simulink library "pv_desoto"  (R2018b)
settings: Solver=VariableStepAuto  StartTime=0.0  StopTime=10.0  RelTol=1e-3
undefined symbols (not defined in the file): Davies, Hay, path_carnot
libraries: carnot x4
settings Model: Creator=P41573  LastModifiedBy=P41573
settings SFSimCC: SimUseLocalCustomCode=off
settings RTWCC: RTWUseLocalCustomCode=off
settings CodeAppCC: StateflowObjectComments=on

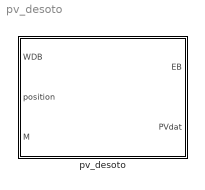
== system pv_desoto ==
  pv_desoto : Subsystem  mask(configurated PV Panel){PathName=fullfile(path_carnot('libsl'), 'Source', 'Electric_Generator', 'pv_desoto', 'parameter_set'), FileName='CEC_sungen_SG-HN100-GG.mat', userPath=on, userParam=on, IL_ref=1.656, alpha_sc=0.001782, a_ref=3.7943, Rs_ref=7.904, Rsh_ref=360.51, I0_ref=1.353e-11, Sref=1000, Tref=25, EgRef=1.121, dEgdT=-0.0002677, KbAngles=[0:5:90], Kb=[1 1 0.9999 0.9996 0.9991 0.9982 0.9965 0.9935 0.9886 0.9807 0.9678 0.9473 0.9148 0.8638 0.7846 0.6644 0.4907 0.2599 0], Kd=0.91, TypeMount=<propagated>, E0=1000, dTc=3, a=-3.348, b=-0.0914, TimeConstant=300, tini=20, ms=1, mp=1}
      mask prompts: PathName "Path"; FileName "Parameter set"; userPath "Edit path and name of parameter set"; userParam "User defined parameters"; IL_ref "reference photo current [A]"; alpha_sc "temperature coef. for Isc [-]"; a_ref "modified diode ideality factor"; Rs_ref "reference serial resistance"; Rsh_ref "reference shunt resistance"; I0_ref "reference saturation current [A]"; Sref "reference irradiance [W/m2]"; Tref "reference cell temperature [°C]"; EgRef "reference band gap [eV]"; dEgdT "temperature dependance of band gap [1/K]"; KbAngles "Kb: angles for longitudinal and transversal IAM [degree]"; Kb "Kb : incident angle modifier beam radiation"; Kd "Kd : Incidence angle modifier diffuse radiation"; TypeMount "Panel type / Mounting Option"; E0 "Reference Irradiation for deltaT (W/m2)"; dTc "SAPM Parameter - deltaT"; a "SAPM Parameter a"; b "SAPM Parameter - b"; TimeConstant "time constant  [s] - (not used)"; tini "initial cell temperature [°C] -(not used)"; ms "Number of modules in series"; mp "Number of modules in parallel"
      mask help:
      | PVPMC (PV-Lib) Single Diode equivalent Model with Sandia temperature model.
      | Parameter tables according to CeC SAMLIB.
      mask init:
      | % [ok, param] = CarnotCallbacks_PvDesotoConf('SetParameters',gcbh,PathName,FileName);
      mask Help: web(fullfile(path_carnot('help'),'pv_desoto.html'),'-helpbrowser')
      mask Callback userPath: [ok, param] = CarnotCallbacks_PvDesoto('UserEdit',gcbh);
      mask Callback userParam: [ok, param] = CarnotCallbacks_PvDesoto('UserEdit',gcbh);
      mask TypeOptions IL_ref: pvl_DeSoto_Sam/IL_ref
      mask TypeOptions alpha_sc: pvl_DeSoto_Sam/alpha_isc
      mask TypeOptions a_ref: pvl_DeSoto_Sam/a_ref
      mask TypeOptions Rs_ref: pvl_DeSoto_Sam/Rs_ref
      mask TypeOptions Rsh_ref: pvl_DeSoto_Sam/Rsh_ref
      mask TypeOptions I0_ref: pvl_DeSoto_Sam/I0_ref
      mask TypeOptions Sref: pvl_DeSoto_Sam/Sref
      mask TypeOptions Tref: pvl_DeSoto_Sam/Tref
      mask TypeOptions EgRef: pvl_DeSoto_Sam/EgRef
      mask TypeOptions dEgdT: pvl_DeSoto_Sam/dEgdT
      mask TypeOptions KbAngles: IAM_Table/angle
      mask TypeOptions Kb: IAM_Table/Kb
      mask TypeOptions Kd: IAM_Table/Kd
      mask TypeOptions TypeMount: <propagated> | Glass/cell/glass - Open rack | Glass/cell/glass - Close roof mount | Glass/cell/polymer sheet - Open rack | Glass/cell/polymer sheet - Insulated back | Polymer/thin-film/steel - Open rack
      mask Callback TypeMount: [ok, param] = CarnotCallbacks_PvDesoto('SetParameters',gcbh);
      mask DialogControl ParameterGroupVar Prompt: Picking a parameter set
      mask DialogControl Control2 Prompt: Carnot public data
      mask DialogControl Control2 Callback: [ok, file] = CarnotCallbacks_PvDesoto('GetFilename',gcbh,'public');
      mask DialogControl Control3 Prompt: Carnot internal data
      mask DialogControl Control3 Callback: [ok, file] = CarnotCallbacks_PvDesoto('GetFilename',gcbh,'internal');
      mask DialogControl Control4 Prompt: Selected path
      mask DialogControl Control4 Callback: [ok, file] = CarnotCallbacks_PvDesoto('GetFilename',gcbh,'selected');
      mask DialogControl Container4 Prompt: Model Parameters
      mask DialogControl Container10 Prompt: PV Panel
      mask DialogControl Container9 Prompt: Optics
      mask DialogControl Container14 Prompt: Temperature Model
      mask DialogControl Container15 Prompt: Array
      mask Display:
      | % user defined picture file
      | picfile = fullfile(path_carnot('intlibsl'), ...
      |         'Source','Electric_Generator','pv_desoto','parameter_set', ...
      |         'pv_desoto.jpg');
      | pic = false;
      | if ~BlockIsInCarnotLibrary    % if not located in library any more
      |     if exist(picfile,'file') % show internal picture if defined
      |         image(imread(picfile), [0.2, 0, 0.6, 1])
      |         set_param(gcb, 'BackgroundColor', 'White')
      |         pic = true;
      |     end
      | end
      | if ~pic    % show public picture
      |     disp('PV-Model\nDesoto')
      |     set_param(gcb, 'BackgroundColor', '[0.5,0.5,1]')
      | end

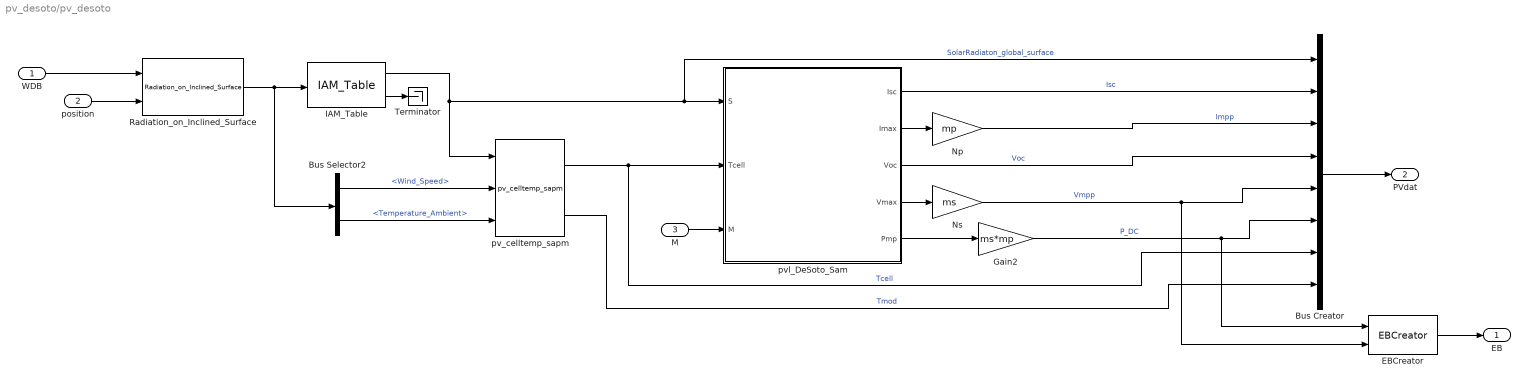
== system pv_desoto/pv_desoto ==
  WDB : Inport
  position : Inport  Port=2
  M : Inport  Port=3
  Bus Creator : BusCreator  Inputs=8
  Bus Selector2 : BusSelector  OutputSignals=Wind_Speed,Temperature_Ambient
  EBCreator : carnot/Basic/Electric/EBCreator  Inport_ID=off  Inport_f=off  Inport_v1=on  Inport_p1=on  Inport_pf1=off  Inport_v2=off  Inport_p2=off  Inport_pf2=off  Inport_v3=off  Inport_p3=off  Inport_pf3=off  ID=2  f=0  v1=0  p1=1e5  pf1=1  v2=0  p2=0  pf2=0  v3=0  p3=0  pf3=0  Annotation_ID=off  Annotation_f=off  Annotation_v1=off  Annotation_p1=off  Annotation_pf1=off  Annotation_v2=off  Annotation_p2=off  Annotation_pf2=off  Annotation_v3=off  Annotation_p3=off  Annotation_pf3=off
      settings: SourceProductName=Carnot
  Gain2 : Gain  Gain=ms*mp
  IAM_Table : carnot/Source/Solar_Thermal/IncidenceAngleModifier/IAM_Table  fta=1  angle=KbAngles  Kb=Kb  Kd=Kd
      settings: SourceProductName=Carnot
  Np : Gain  Gain=mp
  Ns : Gain  Gain=ms
  Radiation_on_Inclined_Surface : carnot/Weather/Radiation_on_Inclined_Surface  sky=Hay-Davies  reflect=0.2
      settings: SourceProductName=Carnot
  Terminator : Terminator
  pv_celltemp_sapm : carnot/Source/Electric_Generator/pv_celltemp_sapm  E0=1000  a=-2.98  b=-0.0471  dTc=2  TypeMount=Glass/cell/glass - Close roof mount  tini=25
      settings: SourceProductName=Carnot
  pvl_DeSoto_Sam : MATLAB Function  TreatAsAtomicUnit=on  mask{IL_ref=IL_ref, alpha_isc=alpha_sc, a_ref=a_ref, Rs_ref=Rs_ref, Rsh_ref=Rsh_ref, I0_ref=I0_ref, Sref=Sref, Tref=Tref, EgRef=EgRef, dEgdT=dEgdT}
      mask prompts: IL_ref "reference photo current [A]"; alpha_isc "temperature coef. for Isc [-]"; a_ref "Modified diode ideality factor"; Rs_ref "Reference serial resistance"; Rsh_ref "reference shunt resistance"; I0_ref "reference saturation current [A]"; Sref "reference irradiance [W/m2]"; Tref "reference cell temperature [°C]"; EgRef "reference band gap [eV]"; dEgdT "temperature dependance of band gap [1/K]"
      mask init:
      | % alpha_isc = panel.alpha_sc;
      | % a_ref = panel.a_ref;
      | % IL_ref = panel.IL_ref;
      | % I0_ref = panel.I0_ref;
      | % Rsh_ref = panel.Rsh_ref;
      | % Rs_ref = panel.Rs_ref;
      | % Sref = panel.Sref;
      | % Tref = panel.Tref;
      | % EgRef = panel.EgRef;
      | % dEgdT = panel.dEgdT;
  EB : Outport
  PVdat : Outport  Port=2
  wires:
  IAM_Table/1 -> pv_celltemp_sapm/1, Bus Creator/1, pvl_DeSoto_Sam/1(S)  "SolarRadiaton_global_surface"
  IAM_Table/2 -> Terminator/1
  pv_celltemp_sapm/1 -> pvl_DeSoto_Sam/2(Tcell), Bus Creator/7  "Tcell"
  Bus Selector2/1 -> pv_celltemp_sapm/2  "<Wind_Speed>"
  pvl_DeSoto_Sam/1(Isc) -> Bus Creator/2  "Isc"
  pvl_DeSoto_Sam/2(Imax) -> Np/1
  pvl_DeSoto_Sam/5(Pmp) -> Gain2/1
  pv_celltemp_sapm/2 -> Bus Creator/8  "Tmod"
  Radiation_on_Inclined_Surface/1 -> Bus Selector2/1, IAM_Table/1
  Bus Selector2/2 -> pv_celltemp_sapm/3  "<Temperature_Ambient>"
  WDB/1 -> Radiation_on_Inclined_Surface/1
  position/1 -> Radiation_on_Inclined_Surface/2
  Ns/1 -> EBCreator/2, Bus Creator/5  "Vmpp"
  Np/1 -> Bus Creator/3  "Impp"
  Gain2/1 -> EBCreator/1, Bus Creator/6  "P_DC"
  pvl_DeSoto_Sam/4(Vmax) -> Ns/1
  pvl_DeSoto_Sam/3(Voc) -> Bus Creator/4  "Voc"
  M/1 -> pvl_DeSoto_Sam/3(M)
  EBCreator/1 -> EB/1
  Bus Creator/1 -> PVdat/1

== matlab function pv_desoto/pvl_DeSoto_Sam ==
  data: Isc output; Imax output; Voc output; Vmax output; S input size=1; Tcell input size=1; M input size=1; IL_ref parameter; Pmp output; alpha_isc parameter; a_ref parameter; Rs_ref parameter; Rsh_ref parameter; I0_ref parameter; Sref parameter size=1; Tref parameter size=1; EgRef parameter size=1; dEgdT parameter size=1
function [Isc, Imax, Voc, Vmax, Pmp] = pvl_DeSoto_Sam(S, Tcell, M, IL_ref, alpha_isc, a_ref, Rs_ref, Rsh_ref, I0_ref, Sref, Tref, EgRef, dEgdT)
% function based on SANDIA-PVPMC Model Library ( https://pvpmc.sandia.gov/ )

%% 1. Calculate corrected Parameters with DeSoto Model
% PVL_CALCPARAMS_DESOTO Applies temperature and irradiance corrections to reference parameters per [1]
% Syntax
%   [IL, I0, Rs, Rsh, nNsVth] = pvl_calcparams_desoto(S, Tcell, alpha_isc, ModuleParameters, EgRef, dEgdt)
%   [IL, I0, Rs, Rsh, nNsVth] = pvl_calcparams_desoto(S, Tcell, alpha_isc, ModuleParameters, EgRef, dEgdt, M)
%   [IL, I0, Rs, Rsh, nNsVth] = pvl_calcparams_desoto(S, Tcell, alpha_isc, ModuleParameters, EgRef, dEgdt, M, Sref)
%   [IL, I0, Rs, Rsh, nNsVth] = pvl_calcparams_desoto(S, Tcell, alpha_isc, ModuleParameters, EgRef, dEgdt, M, Sref, Tref)
%   [IL, I0, Rs, Rsh, nNsVth] = pvl_calcparams_desoto(S, Tcell, alpha_isc, ModuleParameters, EgRef, dEgdt, 'Sref', Sref, 'Tref', Tref)
%
% Description
%   Applies the temperature and irradiance corrections to the IL, I0,
%   Rs, Rsh, and a parameters at reference conditions (IL_ref, I0_ref,
%   etc.) according to the De Soto et. al description given in [1]. The
%   results of this correction procedure may be used in a single diode
%   model to determine IV curves at irradiance = S, cell temperature =
%   Tcell.
%
% Input Parameters:
%   S - The irradiance (in W/m^2) absorbed by the module. S must be >= 0.
%      May be a vector of irradiances, but must be the same size as all
%      other input vectors. Due to a division by S in the script, any S
%      value equal to 0 will be set to 1E-10.
%   Tcell - The average cell temperature of cells within a module in C.
%      Tcell must be >= -273.15. May be a vector of cell temperatures, but
%      must be the same size as all other input vectors.
%   alpha_isc - The short-circuit current temperature coefficient of the
%      module in units of A/C (or A/K).
%   ModuleParameters - a struct with parameters describing PV module
%     performance at reference conditions according to DeSoto's paper. A
%     Parameters may be generated or found by lookup. For ease of use, a library
%     of parameters may be found within the System Advisor Model (SAM) [2].
%     The SAM library has been provided as a .mat file, or may
%     be read and converted into a .mat file by the SAM library reader
%     functions. The ModuleParameters struct must contain (at least) the
%     following 5 fields:
%      ModuleParameters.a_ref - modified diode ideality factor parameter at
%          reference conditions (units of eV), a_ref can be calculated from the
%          usual diode ideality factor (n), number of cells in series (Ns),
%          and cell temperature (Tcell) per equation (2) in [1].
%      ModuleParameters.IL_ref - Light-generated current (or photocurrent)
%          in amperes at reference conditions. This value is referred to
%          as Iph in some literature.
%      ModuleParameters.I0_ref - diode reverse saturation current in amperes,
%          under reference conditions.
%      ModuleParameters.Rsh_ref - shunt resistance under reference conditions (ohms)
%      ModuleParameters.Rs_ref - series resistance under reference conditions (ohms)
%   EgRef - The energy bandgap at reference temperature (in eV). 1.121 eV
%      for silicon. EgRef must be >0.
%   dEgdT - The temperature dependence of the energy bandgap at SRC (in 1/C).
%      May be either a scalar value (e.g. -0.0002677 as in [1]) or a
%      vector of dEgdT values corresponding to each input condition (this
%      may be useful if dEgdT is a function of temperature).
%   M - An optional airmass modifier. If M is given a value of 1,
%      it's assumed absolute (pressure corrected) airmass = 1.5. In this
%      code, M is equal to M/Mref as described in [1] (i.e. Mref is assumed
%      to be 1). Source [1] suggests that an appropriate value for M
%      as a function absolute airmass (AMa) may be:
%      M = polyval([-0.000126, 0.002816, -0.024459, 0.086257, 0.918093], AMa)
%      M may be a vector, but must be of the same size as all other input
%      vectors.
%   Sref - Optional reference irradiance in W/m^2. If omitted, a value of
%      1000 is used.
%   Tref - Optional reference cell temperature in C. If omitted, a value of
%      25 C is used.
%
% Output:
%   IL - Light-generated current in amperes at irradiance=S and
%      cell temperature=Tcell.
%   I0 - Diode saturation curent in amperes at irradiance S and cell temperature Tcell.
%   Rs - Series resistance in ohms at irradiance S and cell temperature Tcell.
%   Rsh - Shunt resistance in ohms at irradiance S and cell temperature Tcell.
%   nNsVth - modified diode ideality factor at irradiance S and cell temperature
%      Tcell. Note that in source [1] nNsVth = a (equation 2). nNsVth is the
%      product of the usual diode ideality factor (n), the number of
%      series-connected cells in the module (Ns), and the thermal voltage
%      of a cell in the module (Vth) at a cell temperature of Tcell.
%
% Notes:
%    If the reference parameters in the ModuleParameters struct are read
%    from a database or library of parameters (e.g. System Advisor Model),
%    it is important to use the same EgRef and dEgdT values that
%    were used to generate the reference parameters, regardless of the
%    actual bandgap characteristics of the semiconductor. For example, in
%    the case of the System Advisor Model library, created as described in
%    [3], EgRef and dEgdT for all modules were 1.121 and -0.0002677,
%    respectively.
%
% Sources:
%
% [1] W. De Soto et al., "Improvement and validation of a model for
%     photovoltaic array performance", Solar Energy, vol 80, pp. 78-88,
%     2006.
%
% [2] System Advisor Model web page. https://sam.nrel.gov.
%
% [3] A. Dobos, "An Improved Coefficient Calculator for the California
%     Energy Commission 6 Parameter Photovoltaic Module Model", Journal of
%     Solar Energy Engineering, vol 134, 2012.
%
% [4] O. Madelung, "Semiconductors: Data Handbook, 3rd ed." ISBN
%     3-540-40488-0
%
% See also
%  This table of reference bandgap energies (EgRef), bandgap energy
%  temperature dependence (dEgdT), and "typical" airmass response (M) is
%  provided purely as reference to those who may generate their own
%  reference module parameters (a_ref, IL_ref, I0_ref, etc.) based upon the
%  various PV semiconductors. Again, we stress the importance of
%  using identical EgRef and dEgdT when generation reference
%  parameters and modifying the reference parameters (for irradiance,
%  temperature, and airmass) per DeSoto's equations.
%  -----------------------------------------------------------------------
%% 2. From DeSoto Parameters calculate Ouputs with Single-Diode Model
% PVL_SINGLEDIODE Solve the single-diode model to obtain a photovoltaic IV curve
%
% Syntax
%   [Result] = pvl_singlediode(IL, I0, Rs, Rsh, nNsVth)
%   [Result] = pvl_singlediode(IL, I0, Rs, Rsh, nNsVth, NumPoints)
%   [Result] = pvl_singlediode(IL, I0, Rs, Rsh, nNsVth, Vpoints)
%
% Description
%   pvl_singlediode solves the single diode equation [1]:
%   I = IL - I0*[exp((V+I*Rs)/(nNsVth))-1] - (V + I*Rs)/Rsh
%   for I and V when given IL, I0, Rs, Rsh, and nNsVth (nNsVth =Ref n*Ns*Vth) which
%   are described later. pvl_singlediode returns a struct which contains
%   the 5 points on the I-V curve specified in SAND2004-3535 [3], and can
%   optionally provide a full IV curve with a user-defined number of
%   points. If all IL, I0, Rs, Rsh, and nNsVth are scalar, a single curve
%   will be returned, if any are vectors (of the same length), multiple IV
%   curves will be calculated.
%
% Input Parameters:
%   IL - Light-generated current (photocurrent) in amperes under desired IV
%      curve conditions. May be a scalar or vector, but vectors must be of
%      same length as all other input vectors.
%   I0 - Diode saturation current in amperes under desired IV curve
%      conditions. May be a scalar or vector, but vectors must be of same
%      length as all other input vectors.
%   Rs - Series resistance in ohms under desired IV curve conditions. May
%      be a scalar or vector, but vectors must be of same length as all
%      other input vectors.
%   Rsh - Shunt resistance in ohms under desired IV curve conditions. May
%      be a scalar or vector, but vectors must be of same length as all
%      other input vectors.
%   nNsVth - the product of three components. 1) The usual diode ideal 
%      factor (n), 2) the number of cells in series (Ns), and 3) the cell 
%      thermal voltage under the desired IV curve conditions (Vth).
%      The thermal voltage of the cell (in volts) may be calculated as 
%      k*Tcell/q, where k is Boltzmann's constant (J/K), Tcell is the
%      temperature of the p-n junction in Kelvin, and q is the elementary 
%      charge of an electron (coulombs). nNsVth may be a scalar or vector, 
%      but vectors must be of same length as all other input vectors.
%   NumPoints - Number of points to compute in each IV curve (optional).
%      Must be a finite scalar value. Non-integer values will be rounded 
%      to the next highest integer (ceil). The default
%      value is 0, resulting in no calculation of IV points other than
%      those specified in [3].
%   Vpoints - number of points, or values of voltage at which to return IV curve points
%      (optional). Must be a scalar, 1d array or a cell array of the same length 
%       as all other input vectors. If a scalar, then the specified number of points
%       is computed for each IV curve.  If a 1d array then points in that array
%       between 0 and Voc are returned for each IV curve.  If a cell array then
%       each element of the cell array contains a 1d array of voltage values
%       at which points are returned.
%
% Output:
%   Result - A structure array with the following fields. All fields have the
%   same number of rows as the largest input vector.
%      Result.Isc - Column vector of short circuit current in amperes.
%      Result.Voc - Column vector of open circuit voltage in volts.
%      Result.Imp - Column vector of current at maximum power point in amperes. 
%      Result.Vmp - Column vector of voltage at maximum power point in volts.
%      Result.Pmp - Column vector of power at maximum power point in watts.
%      Result.Ix - Column vector of current, in amperes, at V = 0.5*Voc.
%      Result.Ixx - Column vector of current, in amperes, at V = 0.5*(Voc+Vmp).
%      Result.V - Cell array of voltages in volts. Element n is an array of 
%        voltages running from V=0 to V=Voc. Voltages are either equally
%        spaced if NumPoints is input, or at values specified in input
%        Vpoints.
%      Result.I - Cell array of currents in amperes. Element n is an array
%        of current values corresponding to the voltage values in element n
%        of Result.V.
%
% Notes:
%    1) The solution employed to solve the implicit diode equation utilizes
%       the Lambert W function to obtain an explicit function of V=f(i) and
%       I=f(V) as shown in [2].
%
% Sources:
%
% [1] S.R. Wenham, M.A. Green, M.E. Watt, "Applied Photovoltaics" 
%     ISBN 0 86758 909 4
%
% [2] A. Jain, A. Kapoor, "Exact analytical solutions of the parameters of 
%     real solar cells using Lambert W-function", Solar Energy Materials 
%     and Solar Cells, 81 (2004) 269-277.
%
% [3] D. King et al, "Sandia Photovoltaic Array Performance Model",
%     SAND2004-3535, Sandia National Laboratories, Albuquerque, NM
%
%% start calculation
if S > 0
    % calc parameters with DeSoto Model
    k = 8.617332478e-5; % Boltzmann constant in units of eV/K    
    Tref_K = Tref + 273.15; % Reference cell temperature in Kelvin
    Tcell_K = Tcell + 273.15; % cell temperature in Kelvin
    
    %These parameters (a, I_L, I_o, M, and R_sh) need to be vectors of equal
    %length to the number of conditions (number of S,Tcell pairs).
    E_g = EgRef.*(1+dEgdT.*(Tcell_K-Tref_K)); % Equation 10 in [1]
    nNsVth = a_ref.*(Tcell_K./Tref_K); % Equation 8 in [1]
    IL = S./Sref.*M.*(IL_ref+alpha_isc.*(Tcell_K-Tref_K));
    % IL(isnan(M) | M<0 | S <= 0) = 0; % If there is no light (or light which generates no current), then no current is produced
    % Equation 9 in [1]
    I0 = I0_ref.*((Tcell_K./Tref_K).^3).*exp((EgRef./(k.*Tref_K))-(E_g./(k*Tcell_K)));
    Rsh = Rsh_ref.*(Sref./S); % Equation 12 in [1]    
    Rs = Rs_ref;
    
    % claculate output with single diode model 
    Isc = I_from_V(Rsh, Rs, nNsVth, 0, I0, IL);% Find Isc using Lambert W    
    Voc = V_from_I(Rsh, Rs, nNsVth, 0, I0, IL);% Find Voc using Lambert W
    % Calculate I, V and P at the maximum power point
    [Imax, Vmax, Pmp] = calc_Pmp_bisect(IL, I0, nNsVth, Rs, Rsh);
    
    % End of code which finds Imax, Vmax, Pmax
else
    Imax = 0*S;
    Pmp = 0*S;
    Vmax = 0*S;
    Voc = 0*S;
    Isc = 0*S;    
end


function V = V_from_I(Rsh, Rs, nNsVth, I, Io, Iphi)

% calculates V from I per Eq 3 Jain and Kapoor 2004
% uses Lambert W implemented in pvl_lambertw

% Generate the argument of the LambertW function
argW = (Io*Rsh/nNsVth) .* ...
    exp(Rsh*(-I+Iphi+Io)/(nNsVth));
inputterm = pvl_lambertw(argW); % Get the LambertW output
f = isnan(inputterm); % If argW is too big, the LambertW result will be NaN and we have to go to logspace

% If it is necessary to go to logspace
if f
    % Calculate the log(argW) if argW is really big
    logargW = log(Io) + log(Rsh) + Rsh.*(Iphi+Io-I)./(nNsVth)...
        - (log(nNsVth));
    % Three iterations of Newton-Raphson method to solve w+log(w)=logargW.
    % The initial guess is w=logargW. Where direct evaluation (above) results
    % in NaN from overflow, 3 iterations of Newton's method gives
    % approximately 8 digits of precision.
    w = logargW;
    for i=1:3
        w = w*((1-log(w)+logargW)/(1+w));
    end
    inputterm = w;
end
% Eqn. 3 in Jain and Kapoor, 2004
V = Rsh*(-I*(Rs/Rsh + 1) + Iphi - nNsVth/Rsh*inputterm + Io);


function I = I_from_V(Rsh, Rs, nNsVth, V, Io, Iphi)
% calculates I from V per Eq 2 Jain and Kapoor 2004
% uses Lambert W implemented in pvl_lambertw

argW = Rs*Io*Rsh*exp(Rsh * (Rs*(Iphi+Io)+V) / (nNsVth*(Rs+Rsh)) ) / (nNsVth * (Rs+Rsh));
inputterm = pvl_lambertw(argW);

% Eqn. 4 in Jain and Kapoor, 2004

I = -V/(Rs + Rsh) - (nNsVth./Rs) * inputterm + ...
    Rsh * (Iphi + Io) / (Rs + Rsh);


function W = calc_phi_exact(Imp, IL, Io, a, Rsh)

% calculates W(phi) where phi is the argument of the
% Lambert W function in V = V(I) at I=Imp ([2], Eq. 3).  Formula for
% phi is given in code below as argw.

% phi
argw = Rsh*Io/a*exp(Rsh*(IL + Io - Imp)/a);

% Screen out any negative values for argw
% take care of any numerical overflow by evaluating log(W(phi))
if argw < 0
    logargW = log(Rsh) + log(Io) - log(a) + Rsh.*(IL + Io - Imp)./a;
    % Three iterations of Newton-Raphson method to solve w+log(w)=logargW.
    % The initial guess is w=logargW. Where direct evaluation (above) results
    % in NaN from overflow, 3 iterations of Newton's method gives
    % approximately 8 digits of precision.
    x = logargW;
    for i=1:5
        x = x*((1-log(x)+logargW)/(1+x));
    end
    W = x;
else
    W = pvl_lambertw(argw);
end


function Imp = calc_Imp_bisect(Iph,Io,a,Rs,Rsh)

% calculates the value of Imp (current at maximum power point) for an IV
% curve with parameters Iph, Io, a, Rs, Rsh.  Imp is found as the value of
% I for which g(I)=dP/dV (I) = 0.

% Set up lower and upper bounds on Imp
A = 0*Iph;
B = Iph+Io;

% Detect when lower and upper bounds are not consistent with finding the
% zero of dP/dV

gA = g(A,Iph,Io,a,Rs,Rsh);
gB = g(B,Iph,Io,a,Rs,Rsh);

if gA*gB > 0
    % where gA*gB > 0, then there is a problem with the IV curve parameters.
    % In the event where gA and gB have the same sign, alert the user with
    % a warning and replace erroneous cases with NaN
    error(['Error: The single diode parameters are such that dP/dV may not have' ...
        ' a zero. A NaN value has been reported.'])
end
% midpoint is initial guess for Imp
p = (A+B)/2;
err = g(p,Iph,Io,a,Rs,Rsh);  % value of dP/dV at initial guess p

while max(abs(B-A))>1e-6   % set precision of estimate of Imp to 1e-6 (A)
    gA = g(A,Iph,Io,a,Rs,Rsh); % value of dP/dV at left endpoint
    if gA*err <0
        B = p;
    else
        A = p;
    end
    p = (A+B)/2;
    %     u = (gA*err) < 0;
    %     B(u) = p(u);
    %     A(~u) = p(~u);
    err = g(p,Iph,Io,a,Rs,Rsh);
end
Imp = p;


function y = g(I,Iph,Io,a,Rs,Rsh)
% calculates dP/dV exactly, using p=I*V=I*V(I), where V=V(I) uses the
% Lambert's W function W(phi) ([2], Eq. 3).
z = calc_phi_exact(I,Iph,Io,a,Rsh);  % calculate W(phi)
% calculate dP/dV
y = (Iph + Io - 2*I)*Rsh - 2*I*Rs - a*z +I*Rsh*z/(1+z);


function [Imp, Vmp, Pmp] = calc_Pmp_bisect(Iph,Io,a,Rs,Rsh)
% Returns Imp, Vmp, Pmp for the IV curve described by input parameters.
% Vectorized.
Imp = calc_Imp_bisect(Iph,Io,a,Rs,Rsh);  % find Imp
z = calc_phi_exact(Imp,Iph,Io,a,Rsh);  % Calculate W(phi) at Imp, where W is Lambert's W function and phi is its argument ([2], Eq. 3)
Vmp = (Iph+Io-Imp)*Rsh - Imp*Rs - a*z;  % Compute V from Imp and W(phi)
Pmp = Vmp*Imp;


function w = pvl_lambertw(z)
%
%
% PVL_LAMBERTW Compute values for the Lambert W Function W(z).
%
% Syntax
%   W = pvl_lambertw(z)
%
% Description
%   W = LAMBERTW(Z) computes the principal value of the Lambert
%   W Function, the solution of Z = W*exp(W).  Z may be a
%   complex scalar or array.  For real Z, the result is real on
%   the principal branch for Z >= -1/e.
%
%   The algorithm uses series approximations as initializations
%   and Halley's method as developed in Corless, Gonnet, Hare,
%   Jeffrey, Knuth, "On the Lambert W Function", Advances in
%   Computational Mathematics, volume 5, 1996, pp. 329-359.

%   Original code by Pascal Getreuer 2005-2006, modified by
%   Didier Clamond, 2005.  Code downloaded from
%   http://www.getreuer.info/home/lambertw and modified for inclusion in
%   PVLib.
%
%   Matlab includes a lambertw.m function using a very similar algorithm
%   in the Symbolic Math Toolbox.
%
% Inputs:
%       Z - scalar or vector of values at which W(Z) will be evaluated.
%
% Outputs:
%       w - scalar or vector of values of W(Z) on the principal branch.
%
% Sources:
%
%   [1] R.M. Corless, G.H. Gonnet, D.E.G. Hare, G.J. Jeffery, and D.E.
%       Knuth. "On the Lambert W Function." Advances in Computational
%       Mathematics, vol. 5, 1996

% Use asymptotic expansion w = log(z) - log(log(z)) for most z
tmp = log(z + (z == 0));

% Use a series expansion when close to the branch point -1/e
k = (abs(z + 0.3678794411714423216) <= 1.5);
if k
    tmp = sqrt(5.43656365691809047*z + 2) - 1; % [1], Eq. 4.22 and text
    w = tmp;
else
    w = tmp - log(tmp + (tmp == 0));
end
for k = 1:36
    % Converge with Halley's method ([1], Eq. 5.9), about 5 iterations satisfies
    % the tolerance for most z
    c1 = exp(w);
    c2 = w*c1 - z;
    w1 = w + (w ~= -1);
    dw = c2/(c1*w1 - ((w + 2)*c2./(2*w1)));
    w = w - dw;
    if all(abs(dw) < 0.7e-16*(2+abs(w)))
        break;
    end
end
